simulink model "batterymonitoringsystem"  (R2023a)
settings: Solver=ode23tb  StartTime=0.0  StopTime=1000.0  RelTol=1e-3
undefined symbols (not defined in the file): Ion, Lithium
libraries: spsBatteryLib x1, spsBreakerLib x1, spsControlledCurrentSourceLib x1, spsDCVoltageSourceLib x1, spsDiodeLib x1, spsGroundLib x1, spsIdealSwitchLib x1, spsSeriesRLCBranchLib x1, spsVoltageMeasurementLib x1, sps_lib x1
settings Model: Creator=Asus  LastModifiedBy=Asus

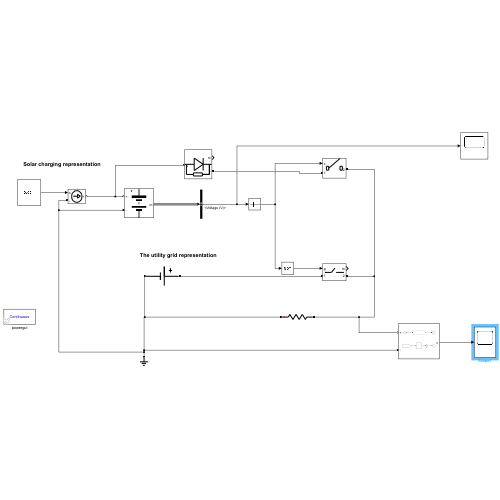
[thumbnail: Simulink's stored preview of the top-level diagram]
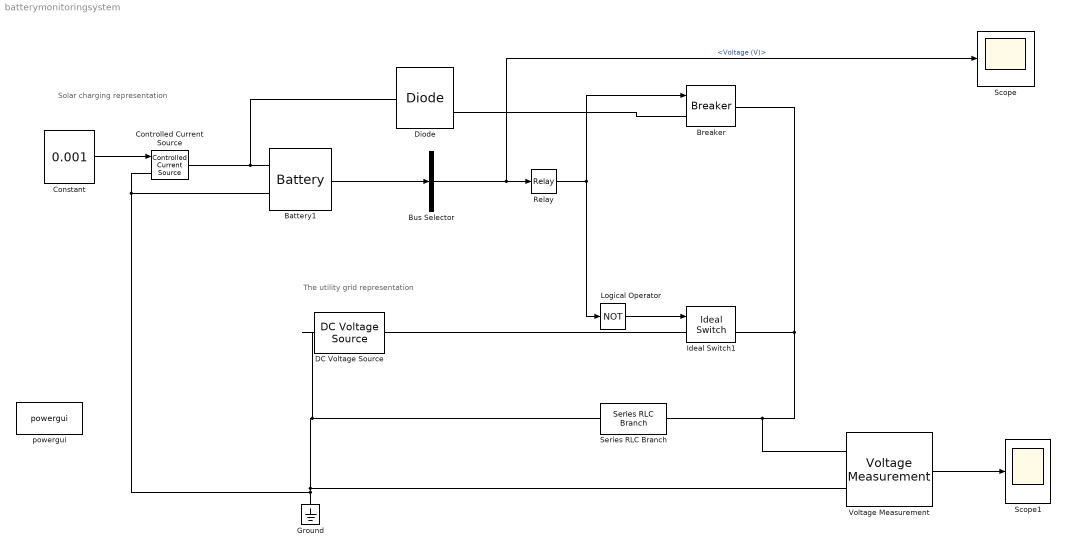
== system batterymonitoringsystem ==
  note: The utility grid representation
  note: Solar charging representation
  Battery1 : spsBatteryLib/Battery  BatType=Lithium-Ion  ShowTempParam=off  ThermalPreset=no  ShowAgeParam=off  NomV=5  NomQ=0.01  SOC=100  Batt_Tr=100  PresetModel=on  MaxQ=0.01  MinV=3.75  FullV=5.8199  Dis_rate=0.0043478  R=5  Normal_OP=0.0090435  expZone="[5.4019   0.0004913]"  current=[6.5 13 32.5]  Units=Time  Tci=20  NomT=20  T2=-30  MaxQ2=4.8  FullV2=7.1  Normal_OP2=5.655  expZone2="[6.58           1]"  Rca=0.6  ti=2000  Dp=0  Neq0=0  Tsim=1e6  Ta1=25  Qeol=5.4*0.9  Reol=0.013333*1.2  Char_age=[2.3478, 3]  Dis_age=[2.3478, 10]  N1=1500  N2=10500  N3=1000  N4=1400  Ta2=45  N5=950
  Breaker : spsBreakerLib/Breaker  InitialState=0  SwitchingTimes="[1/60  5/60]"  External=on  BreakerResistance=0.01  SnubberResistance=inf  SnubberCapacitance=0  Measurements=None  MoreParameters=on  NoBreakLoop=off
  Bus Selector : BusSelector  OutputSignals=Voltage (V)
  Constant : Constant  Value=0.001
  Controlled Current Source : spsControlledCurrentSourceLib/Controlled Current Source  Initialize=off  Source_Type=DC  Amplitude=0  Phase=0  Frequency=0  Measurements=None
  DC Voltage Source : spsDCVoltageSourceLib/DC Voltage Source  Amplitude=5  Measurements=None
  Diode : spsDiodeLib/Diode  Ron=0.1  Lon=0  Vf=0.8  IC=0  UseSnubber=0  Rs=500  Cs=250e-9  Measurements=on
  Ground : spsGroundLib/Ground  LConnTagsString=a
  Ideal Switch1 : spsIdealSwitchLib/Ideal Switch  Ron=0.001  Lon=0  IC=0  Rs=inf  Cs=0  Measurements=on
  Logical Operator : Logic  Operator=NOT  AllPortsSameDT=off  OutDataTypeStr=boolean
  Relay : Relay  OnSwitchValue=5  OffSwitchValue=3.5
  Scope : Scope
  Scope1 : Scope
  Series RLC Branch : spsSeriesRLCBranchLib/Series RLC Branch  LConnTagsString=__new0  RConnTagsString=__new0  BranchType=R  Resistance=100  Inductance=1e-3  SetiL0=off  InitialCurrent=0  Capacitance=1e-6  Setx0=off  InitialVoltage=0  Measurements=None
  Voltage Measurement : spsVoltageMeasurementLib/Voltage Measurement  PhasorSimulation=off  OutputType=Complex  PSBequivalent=0
  powergui : sps_lib/powergui  Priority=1  SimulationMode=Continuous  SampleTime=50e-6  frequency=60  Iterations=50  frequencyindice=0  Pbase=100e6  ErrMax=1e-4  UnitsV=kV  UnitsW=MW  buscounter=0  FunctionMessages=off  echomessages=off  EnableUseOfTLC=off  CurrentSourceSwitches=off  DisableSnubberDevices=off  DisableRonSwitches=off  DisableVfSwitches=off  DisplayEquations=off  AutomaticDiscreteSolvers=off  SolverType=Tustin/Backward Euler (TBE)  Interpol=off  ExternalGateDelay=off  methode=off  Ts=100  x0status=blocks  SPID=on  SwTol=0  HookPort=off  NonlinearTolerance=1e-4  nMaxIteration=100  ContinueOnMaxIteration=off  RestoreLinks=warning  ResistiveCurrentMeasurement=off  Frange=[0:2:500]  Ylog=off  Xlog=on  ShowGrid=off  save=off  variable=ZData  structure=0  ZoomFFT=off  StartTime=0.0  cycles=1  DisplayStyle=1  fundamental=60  FreqAxis=off  MaxFrequency=1000  frequencyindicesteady=1  RmsSteady=1  display=off
  wires:
  Constant/1 -> Controlled Current Source/1
  Battery1/1 -> Bus Selector/1
  Bus Selector/1 -> Scope/1, Relay/1  "<Voltage (V)>"
  Relay/1 -> Breaker/1, Logical Operator/1
  Logical Operator/1 -> Ideal Switch1/1
  Voltage Measurement/1 -> Scope1/1
  connections:
  Controlled Current Source/RConn1 -- Diode/LConn1 -- Battery1/LConn1
  DC Voltage Source/RConn1 -- Ideal Switch1/LConn1
  Ideal Switch1/RConn1 -- Voltage Measurement/LConn1 -- Series RLC Branch/RConn1 -- Breaker/RConn1
  Controlled Current Source/LConn1 -- Battery1/LConn2 -- Series RLC Branch/LConn1 -- DC Voltage Source/LConn1 -- Voltage Measurement/LConn2 -- Ground/LConn1
  Diode/RConn1 -- Breaker/LConn1
